simulink model "simuRLC"  (R2022b)
settings: Solver=VariableStepAuto  StartTime=0.0  StopTime=0.04  MaxStep=1e-6  RelTol=1e-3
values from neighbouring files (symbols this model uses):
  C = 1e-3    (= 0.001)    [RLCdynamics.m]    (also in simulateRLC.m)
  L = 1e-3    (= 0.001)    [RLCdynamics.m]    (also in simulateRLC.m)
  R = 2    [RLCdynamics.m]    (also in simulateRLC.m)
settings Model: Creator=sooru  LastModifiedBy=sooru

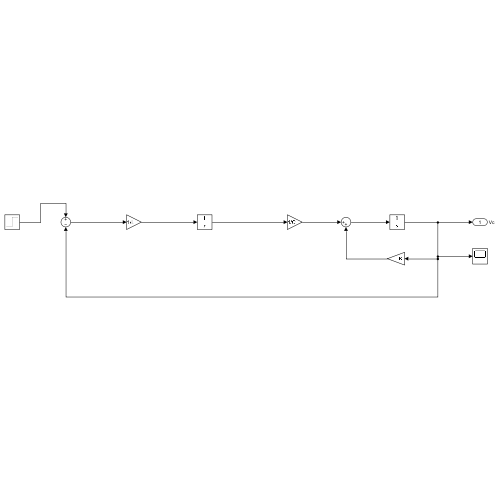
[thumbnail: Simulink's stored preview of the top-level diagram]
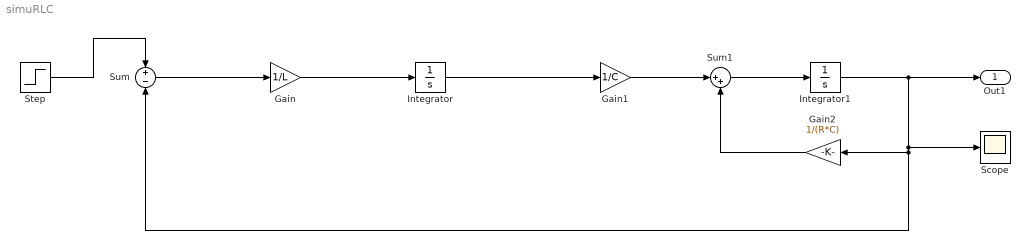
== system simuRLC ==
  Gain : Gain  Gain=1/L
  Gain1 : Gain  Gain=1/C
  Gain2 : Gain  Gain=1/(R*C)
  Integrator : Integrator
  Integrator1 : Integrator
  Scope : Scope
  Step : Step  Time=0  SampleTime=0
  Sum : Sum  Inputs=+-
  Sum1 : Sum  Inputs=|++
  Out1 : Outport  SignalName=Vc
  wires:
  Step/1 -> Sum/1
  Sum/1 -> Gain/1
  Gain/1 -> Integrator/1
  Integrator/1 -> Gain1/1
  Gain1/1 -> Sum1/1
  Sum1/1 -> Integrator1/1
  Integrator1/1 -> Sum/2, Gain2/1, Scope/1, Out1/1
  Gain2/1 -> Sum1/2
